simulink subsystem "TB66FNG"  (R2024a)
settings: Solver=VariableStepAuto  StartTime=0.0  StopTime=10.0  RelTol=1e-3
libraries: stm32f4xxblockslib x4
settings Model: Creator=Peter  LastModifiedBy=Peter

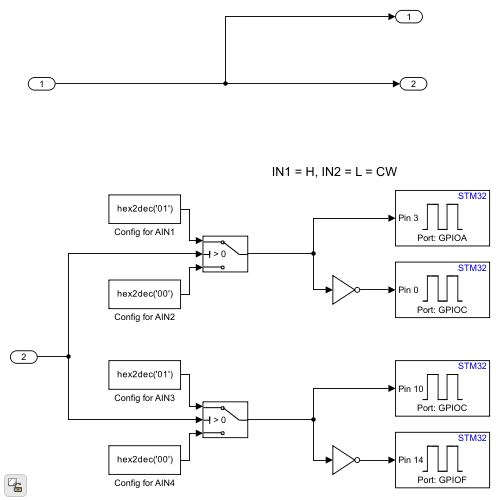
[thumbnail: Simulink's stored preview of the top-level diagram]
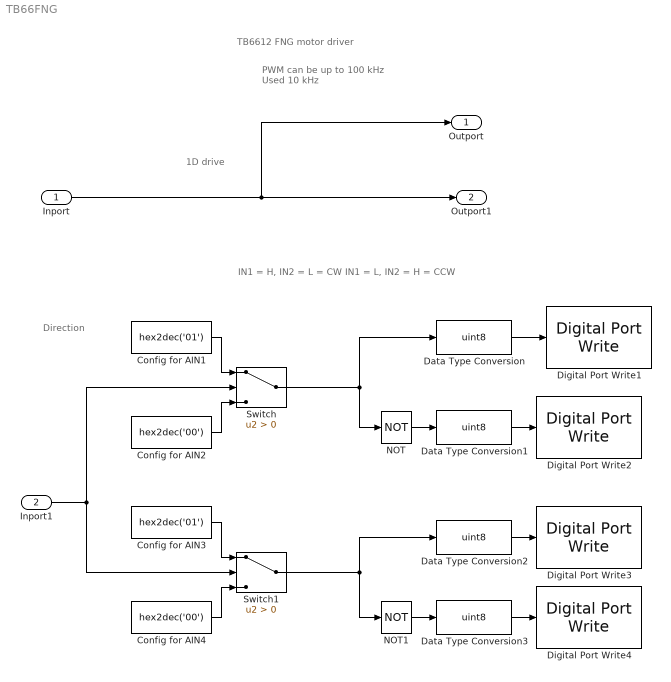
== system TB66FNG ==
  note: PWM can be up to 100 kHz
      | Used 10 kHz
  note: TB6612 FNG motor driver
  note: 1D drive
  note: Direction
  note: IN1 = H, IN2 = L = CW
      | IN1 = L, IN2 = H = CCW
  Inport : Inport
  Inport1 : Inport  Port=2
  Config for AIN1 : Constant  Value=hex2dec('01')  OutDataTypeStr=uint8
  Config for AIN2 : Constant  Value=hex2dec('00')  OutDataTypeStr=uint8
  Config for AIN3 : Constant  Value=hex2dec('01')  OutDataTypeStr=uint8
  Config for AIN4 : Constant  Value=hex2dec('00')  OutDataTypeStr=uint8
  Data Type Conversion{,1..3} (4 alike) : DataTypeConversion  OutDataTypeStr=uint8  SaturateOnIntegerOverflow=off  RndMeth=Floor
  Digital Port Write1 : stm32f4xxblockslib/Digital Port Write  PortName=GPIOA  PinNumber=[3]  ReadOperation=off  IOAsArray=off  EnableSimPort=off  hoistedMaskSrc=ECSoC/ECSimCodegen/Digital Port Write
      settings: LibrarySourceBlock=stm32f7xxblockslib/Digital Port Write
  Digital Port Write2 : stm32f4xxblockslib/Digital Port Write  PortName=GPIOC  PinNumber=[0]  ReadOperation=off  IOAsArray=off  EnableSimPort=off  hoistedMaskSrc=ECSoC/ECSimCodegen/Digital Port Write
      settings: LibrarySourceBlock=stm32f7xxblockslib/Digital Port Write
  Digital Port Write3 : stm32f4xxblockslib/Digital Port Write  PortName=GPIOC  PinNumber=[10]  ReadOperation=off  IOAsArray=off  EnableSimPort=off  hoistedMaskSrc=ECSoC/ECSimCodegen/Digital Port Write
      settings: LibrarySourceBlock=stm32f7xxblockslib/Digital Port Write
  Digital Port Write4 : stm32f4xxblockslib/Digital Port Write  PortName=GPIOF  PinNumber=[14]  ReadOperation=off  IOAsArray=off  EnableSimPort=off  hoistedMaskSrc=ECSoC/ECSimCodegen/Digital Port Write
      settings: LibrarySourceBlock=stm32f7xxblockslib/Digital Port Write
  NOT : Logic  Operator=NOT  IconShape=distinctive  AllPortsSameDT=off  OutDataTypeStr=boolean
  NOT1 : Logic  Operator=NOT  IconShape=distinctive  AllPortsSameDT=off  OutDataTypeStr=boolean
  Switch : Switch  Criteria=u2 > Threshold  SaturateOnIntegerOverflow=off  InputSameDT=off
  Switch1 : Switch  Criteria=u2 > Threshold  SaturateOnIntegerOverflow=off  InputSameDT=off
  Outport : Outport
  Outport1 : Outport  Port=2
  wires:
  Config for AIN1/1 -> Switch/1
  Config for AIN2/1 -> Switch/3
  Switch/1 -> NOT/1, Data Type Conversion/1
  Inport1/1 -> Switch/2, Switch1/2
  Config for AIN4/1 -> Switch1/3
  Config for AIN3/1 -> Switch1/1
  Switch1/1 -> Data Type Conversion2/1, NOT1/1
  NOT/1 -> Data Type Conversion1/1
  NOT1/1 -> Data Type Conversion3/1
  Inport/1 -> Outport/1, Outport1/1
  Data Type Conversion/1 -> Digital Port Write1/1
  Data Type Conversion1/1 -> Digital Port Write2/1
  Data Type Conversion2/1 -> Digital Port Write3/1
  Data Type Conversion3/1 -> Digital Port Write4/1
